simulink model "MSE_SIMULINKS"  (R2016b)
settings: Solver=VariableStepDiscrete  StartTime=0.0  StopTime=inf  RelTol=1e-3
values from neighbouring files (symbols this model uses):
  D = posMSED    [MSE_matlab2.m]    (also in adaptive_equalization.m; channel_coding_matlab.m = sum(C,2))
  gk = gk/Kg    [MSE_matlab2.m]    (also in adaptive_equalization.m)
  M = 8    [ML_receiver_matlab.m]    (also in MSE_matlab2.m = 16; OFDM1.m = 64; adaptive_equalization.m = 16)
libraries: commchan3 x1, commrandsrc3 x1, commdigbbndam3 x1, dspstat3 x1
settings Model: Creator=Shu  LastModifiedBy=Shu
settings DataIOCC: LimitDataPoints=on  SaveOutput=off  SaveTime=off
settings OptimizationCC: BooleanDataType=off  DefaultParameterBehavior=Inlined  LocalBlockOutputs=off  LifeSpan=inf
settings DebuggingCC: AlgebraicLoopMsg=error  SingleTaskRateTransMsg=error  AllowSymbolicDim=off  SFUnexpectedBacktrackingDiag=warning  SFNoUnconditionalDefaultTransitionDiag=warning  SFExecutionAtInitializationDiag=none
settings GRTTargetCC: TargetLangStandard=C89/C90 (ANSI)  GeneratePreprocessorConditionals=Disable all
settings ConfigComp: CovMetricSettings=dw  CovHtmlReporting=on  CovSaveCumulativeToWorkspaceVar=on  CovSaveSingleToWorkspaceVar=on  CovExternalEMLEnable=off  CovSFcnEnable=off

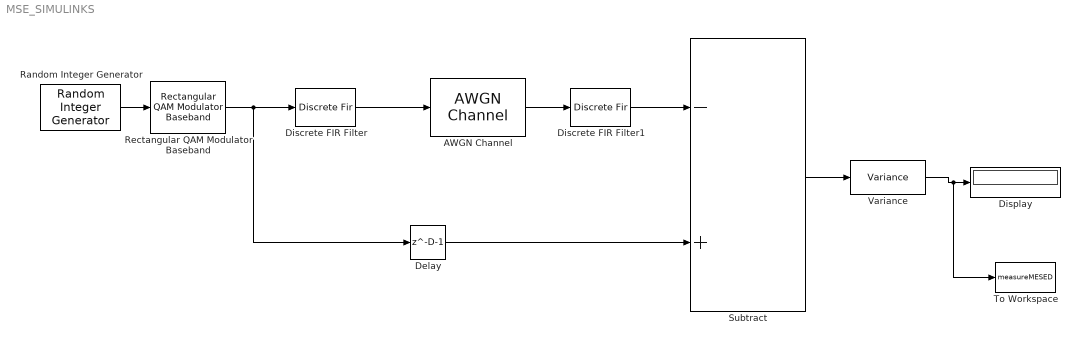
== system MSE_SIMULINKS ==
  AWGN Channel : commchan3/AWGN Channel  InputProcessing=Columns as channels (frame based)  seed=67  noiseMode="Signal to noise ratio  (SNR)"  EbNodB=10  EsNodB=10  SNRdB=SNRdB  bitsPerSym=1  Ps=2*(M-1)/3  Tsym=1  variance=1
  Delay : Delay  DelayLength=D-1  InitialCondition=0
  Discrete FIR Filter : DiscreteFir  Coefficients=gk  InputProcessing=Columns as channels (frame based)
  Discrete FIR Filter1 : DiscreteFir  Coefficients=coptD.'  InputProcessing=Columns as channels (frame based)
  Display : Display
  Random Integer Generator : commrandsrc3/Random Integer Generator  SetSize=M  SeedSource=Auto  Seed=0  SampleTime=1  SamplesPerFrame=1  OutputDataType=double  SimulateUsing=Interpreted execution
  Rectangular QAM Modulator Baseband : commdigbbndam3/Rectangular QAM Modulator Baseband  M=M  InType=Integer  Enc=Gray  Mapping=[0:15]  PowType=Min. distance between symbols  MinDist=2  AvgPow=1  PeakPow=1  Ph=0  outDtype=double  outWordLen=16  outUDDataType=sfix(16)  outFracLenMode=Best precision  outFracLen=15  outDataTypeStr=double  outLastDataTypeStr=double
  Subtract : Sum  Inputs=-+
  To Workspace : ToWorkspace  VariableName=measureMESED  SampleTime=-1
      settings: MaxDataPoints=1
  Variance : dspstat3/Variance  run=on  reset_popup=None  InputProcessing=Columns as channels (frame based)  directionMode=Each column  dimension=1  roiEnable=off  roiType=Rectangles  roiPortion=Entire ROI  roiOutput=Individual statistics for each ROI  roiFlag=off  roundingMode=Floor  overflowMode=off
  wires:
  Random Integer Generator/1 -> Rectangular QAM Modulator Baseband/1
  Rectangular QAM Modulator Baseband/1 -> Delay/1, Discrete FIR Filter/1
  Discrete FIR Filter/1 -> AWGN Channel/1
  AWGN Channel/1 -> Discrete FIR Filter1/1
  Discrete FIR Filter1/1 -> Subtract/1
  Delay/1 -> Subtract/2
  Subtract/1 -> Variance/1
  Variance/1 -> To Workspace/1, Display/1
